simulink model "Likitha_Version_3_1"  (R2025b)
settings: Solver=VariableStepAuto  StartTime=0.0  StopTime=0.3  RelTol=1e-3
undefined symbols (not defined in the file): Ion, Lithium
libraries: spsBatteryLib x50, spsSeriesRLCBranchLib x15, spsCurrentMeasurementLib x10, spsVoltageMeasurementLib x10, spsIdealSwitchLib x9, spsMosfetLib x7, slpidlib x4, spsPWMGeneratorDCDCLib x2, spspowerguiLib x2, spsACVoltageSourceLib x1, eeHysteresisControl x1, spsDCMachineLib x1
(part 1 of 3)
settings Model: Creator=Jatay  LastModifiedBy=Jatay

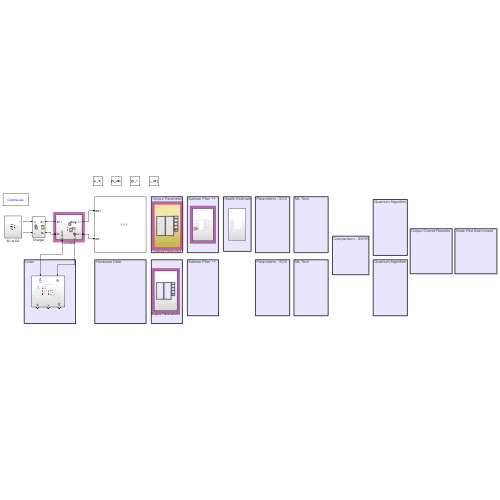
[thumbnail: Simulink's stored preview of the top-level diagram]
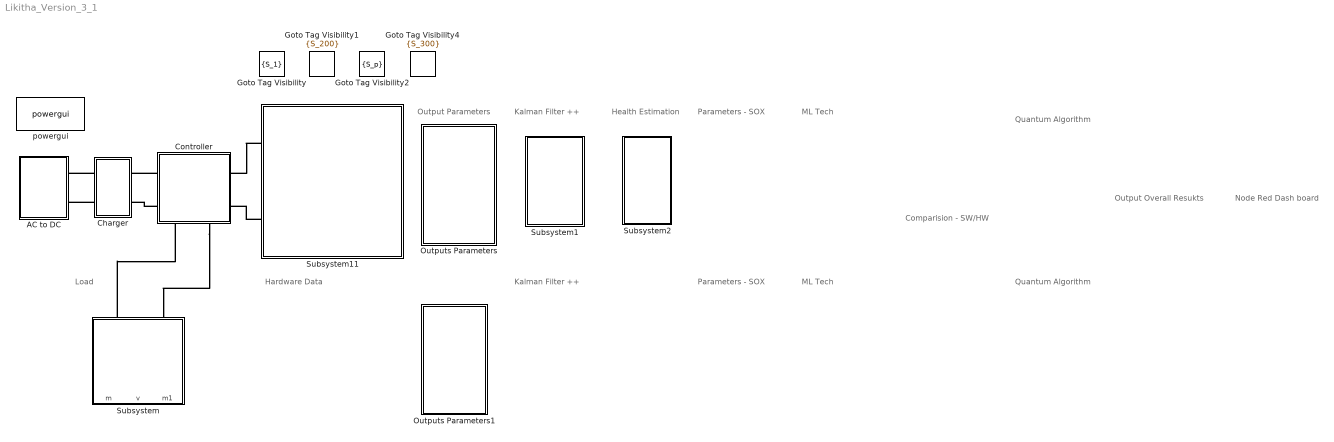
== system Likitha_Version_3_1 ==
  note: Health Estimation
  note: Output Parameters
  note: Hardware Data
  note: Kalman Filter ++
  note: Parameters - SOX
  note: ML Tech
  note: Kalman Filter ++
  note: Parameters - SOX
  note: ML Tech
  note: Comparision - SW/HW
  note: Quantum Algorithm
  note: Quantum Algorithm
  note: Output Overall Resukts
  note: Node Red Dash board
  note: Load
  AC to DC : Subsystem
  Charger : Subsystem
  Controller : Subsystem
      settings: PortSchema="{\"entries\":[{\"content\":{\"sides\":[{\"content\":{\"connectorIds\":[\"LConn1\",\"LConn2\"]},\"type\":\"ConnectorPlacement.EquallySpacedRectSide\",\"uuid\":\"ff826bc9-6c6d-4d1b-bda7-2b84bf27e69f\"},{\"content\":{\"connectorIds\":[\"RConn1\",\"RConn2\"],\"side\":\"RIGHT\"},\"type\":\"ConnectorPlacement.EquallySpacedRectSide\",\"uuid\":\"011d9e86-4a41-4c7c-aeec-abd747732ee3\"},{\"content\":{\"side\":\"TOP\"},\"type\":\"ConnectorPlacement.EquallySpacedRectSide\",\"uuid\":\"d78c1a77-7558-4fb8-9c60-436806204744\"},{\"content\":{\"connectorIds\":[\"RConn3\",\"RConn4\"],\"side\":\"BOTTOM\"},\"type\":\"ConnectorPlacement.EquallySpacedRectSide\",\"uuid\":\"cc43dd25-8365-4f89-92e1-f58595e4ba76\"}]},\"type\":\"ConnectorPlacement.EquallySpacedConnector\",\"uuid\":\"01dac08a-c3c2-418e-8901-b9ec60af109b\"}],\"packageUris\":[\"http://schema.mathworks.com/mf0/Connector/R2020b\"],\"version\":\"1.0\"}"
  Goto Tag Visibility : GotoTagVisibility  GotoTag=S_1
  Goto Tag Visibility1 : GotoTagVisibility  GotoTag=S_200
  Goto Tag Visibility2 : GotoTagVisibility  GotoTag=S_p
  Goto Tag Visibility4 : GotoTagVisibility  GotoTag=S_300
  Outputs Parameters : Subsystem
  Outputs Parameters1 : Subsystem
  Subsystem : Subsystem
  Subsystem1 : Subsystem
  Subsystem11 : Subsystem
      mask Display: image('swapping.webp');
  Subsystem2 : Subsystem
  powergui : spspowerguiLib/powergui  Priority=1  SimulationMode=Continuous  SampleTime=50e-6  frequency=60  Iterations=50  frequencyindice=0  Pbase=100e6  ErrMax=1e-4  UnitsV=kV  UnitsW=MW  buscounter=0  FunctionMessages=off  echomessages=off  EnableUseOfTLC=off  CurrentSourceSwitches=off  DisableSnubberDevices=off  DisableRonSwitches=off  DisableVfSwitches=off  DisplayEquations=off  AutomaticDiscreteSolvers=off  SolverType=Tustin/Backward Euler (TBE)  Interpol=off  ExternalGateDelay=off  methode=off  Ts=100  x0status=blocks  SPID=on  SwTol=0  HookPort=off  NonlinearTolerance=1e-4  nMaxIteration=100  ContinueOnMaxIteration=off  RestoreLinks=warning  ResistiveCurrentMeasurement=off  Frange=[0:2:500]  Ylog=off  Xlog=on  ShowGrid=off  save=off  variable=ZData  structure=0  ZoomFFT=off  StartTime=0.0  cycles=1  DisplayStyle=1  fundamental=60  FreqAxis=off  MaxFrequency=1000  frequencyindicesteady=1  RmsSteady=1  display=off
  connections:
  Charger/LConn1 -- AC to DC/RConn1
  Charger/LConn2 -- AC to DC/RConn2
  Controller/LConn1 -- Charger/RConn1
  Controller/LConn2 -- Charger/RConn2
  Subsystem11/LConn1 -- Controller/RConn1
  Subsystem11/LConn2 -- Controller/RConn2
  Subsystem/LConn1 -- Controller/RConn3
  Controller/RConn4 -- Subsystem/LConn2

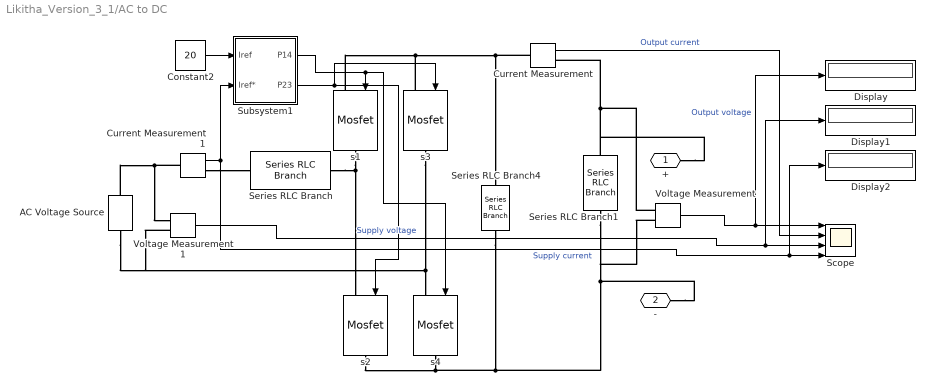
== system Likitha_Version_3_1/AC to DC ==
  AC Voltage Source : spsACVoltageSourceLib/AC Voltage Source  Amplitude=230*sqrt(2)  Phase=0  Frequency=50  SampleTime=0  Measurements=None  BusType=swing  Pref=10e3  Qref=0  Qmin=-inf  Qmax=+inf
  Constant2 : Constant  Value=20
  Current Measurement : spsCurrentMeasurementLib/Current Measurement  PhasorSimulation=off  OutputType=Complex  PSBequivalent=0
  Current Measurement1 : spsCurrentMeasurementLib/Current Measurement  PhasorSimulation=off  OutputType=Complex  PSBequivalent=0
  Display : Display
  Display1 : Display
      settings: Format=short_e
  Display2 : Display
  Scope : Scope  NumInputPorts=4
      settings: ActiveDisplayYMinimum=0  ActiveDisplayYMaximum=500
  Series RLC Branch : spsSeriesRLCBranchLib/Series RLC Branch  LConnTagsString=__new0  RConnTagsString=__new0  BranchType=L  Resistance=1  Inductance=10e-3  SetiL0=off  InitialCurrent=0  Capacitance=1e-6  Setx0=off  InitialVoltage=0  Measurements=None
  Series RLC Branch1 : spsSeriesRLCBranchLib/Series RLC Branch  LConnTagsString=__new0  RConnTagsString=__new0  BranchType=R  Resistance=1  Inductance=10e-3  SetiL0=off  InitialCurrent=0  Capacitance=1e-6  Setx0=off  InitialVoltage=0  Measurements=None
  Series RLC Branch4 : spsSeriesRLCBranchLib/Series RLC Branch  LConnTagsString=__new0  RConnTagsString=__new0  BranchType=C  Resistance=1  Inductance=1e-3  SetiL0=off  InitialCurrent=0  Capacitance=5000e-6  Setx0=off  InitialVoltage=0  Measurements=None
  Subsystem1 : Subsystem
  Voltage Measurement : spsVoltageMeasurementLib/Voltage Measurement  PhasorSimulation=off  OutputType=Complex  PSBequivalent=0
  Voltage Measurement1 : spsVoltageMeasurementLib/Voltage Measurement  PhasorSimulation=off  OutputType=Complex  PSBequivalent=0
  s{1..4} (4 alike) : spsMosfetLib/Mosfet  Ron=0.1  Lon=0  Rd=0.01  Vfd=0  IC=0  Rs=1e5  Cs=inf  Measurements=off
  + : PMIOPort  Side=Right
  - : PMIOPort  Port=2  Side=Right
  wires:
  Current Measurement1/1 -> Display2/1, Scope/4, Subsystem1/2(Iref*)  "Supply current"
  Voltage Measurement/1 -> Display/1, Scope/1  "Output voltage"
  Voltage Measurement1/1 -> Display1/1, Scope/3  "Supply voltage"
  Subsystem1/1("P14 ") -> s4/1, s1/1
  Current Measurement/1 -> Scope/2  "Output current"
  Subsystem1/2(P23) -> s3/1, s2/1
  Constant2/1 -> Subsystem1/1(Iref)
  connections:
  Current Measurement1/LConn1 -- Voltage Measurement1/LConn1 -- AC Voltage Source/RConn1
  Voltage Measurement/LConn1 -- Current Measurement/RConn1 -- Series RLC Branch1/LConn1 -- +/RConn1
  s3/RConn1 -- AC Voltage Source/LConn1 -- Voltage Measurement1/LConn2 -- s4/LConn1
  s2/RConn1 -- s4/RConn1 -- Series RLC Branch4/RConn1 -- Series RLC Branch1/RConn1 -- Voltage Measurement/LConn2 -- -/RConn1
  s1/RConn1 -- s2/LConn1 -- Series RLC Branch/RConn1
  s1/LConn1 -- Current Measurement/LConn1 -- Series RLC Branch4/LConn1 -- s3/LConn1
  Current Measurement1/RConn1 -- Series RLC Branch/LConn1

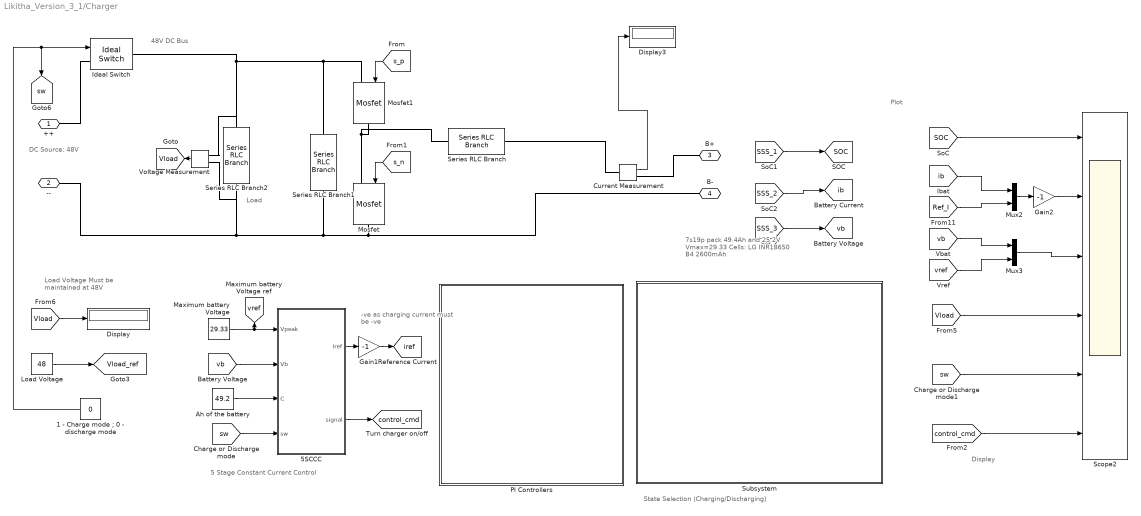
== system Likitha_Version_3_1/Charger ==
  note: Load Voltage
      | Must be
      | maintained at 48V
  note: 48V DC Bus
  note: DC Source:
      | 48V
  note: 7s19p pack
      | 49.4Ah and 25.2V
      | Vmax=29.33
      | Cells:
      | LG INR18650 B4 2600mAh
  note: Plot
  note: -ve as charging
      | current must be -ve
  note: 5 Stage Constant Current Control
  note: Display
  note: Load
  note: State Selection (Charging/Discharging)
  "1 - Charge mode ; 0 - discharge mode  " : Constant  Value=0
  5SCCC : Stateflow chart  TreatAsAtomicUnit=on
  Ah of the battery : Constant  Value=49.2
  Current Measurement : spsCurrentMeasurementLib/Current Measurement  PhasorSimulation=off  OutputType=Complex  PSBequivalent=0
  Display : Display
  Display3 : Display
  Gain1 : Gain  Gain=-1
  Gain2 : Gain  Gain=-1
  Ideal Switch : spsIdealSwitchLib/Ideal Switch  Ron=0.001  Lon=0  IC=0  Rs=1e5  Cs=inf  Measurements=off
  Load Voltage : Constant  Value=48
  Maximum battery Voltage : Constant  Value=29.33
  Mosfet : spsMosfetLib/Mosfet  Ron=0.1  Lon=0  Rd=0.01  Vfd=0  IC=0  Rs=1e5  Cs=inf  Measurements=off
  Mosfet1 : spsMosfetLib/Mosfet  Ron=0.1  Lon=0  Rd=0.01  Vfd=0  IC=0  Rs=1e5  Cs=inf  Measurements=off
  Mux2 : Mux  Inputs=2
  Mux3 : Mux  Inputs=2
  PI Controllers : Subsystem
  Scope2 : Scope  NumInputPorts=6
      settings: Title=SoC  ActiveDisplayYMinimum=96.96249  ActiveDisplayYMaximum=97.0551  DataLoggingVariableName=ScopeData2
  Series RLC Branch : spsSeriesRLCBranchLib/Series RLC Branch  LConnTagsString=__new0  RConnTagsString=__new0  BranchType=RL  Resistance=0.05  Inductance=5.76e-4  SetiL0=off  InitialCurrent=0  Capacitance=1e-6  Setx0=off  InitialVoltage=0  Measurements=None
  Series RLC Branch1 : spsSeriesRLCBranchLib/Series RLC Branch  LConnTagsString=__new0  RConnTagsString=__new0  BranchType=RC  Resistance=0.001  Inductance=5.76e-4  SetiL0=off  InitialCurrent=0  Capacitance=1000e-6  Setx0=off  InitialVoltage=0  Measurements=None
  Series RLC Branch2 : spsSeriesRLCBranchLib/Series RLC Branch  LConnTagsString=__new0  RConnTagsString=__new0  BranchType=R  Resistance=6  Inductance=5.76e-4  SetiL0=off  InitialCurrent=0  Capacitance=1000e-6  Setx0=off  InitialVoltage=0  Measurements=None
  Subsystem : Subsystem
  Voltage Measurement : spsVoltageMeasurementLib/Voltage Measurement  PhasorSimulation=off  OutputType=Complex  PSBequivalent=0
  ++ : PMIOPort  Side=Left
  -- : PMIOPort  Port=2  Side=Left
  B+ : PMIOPort  Port=3  Side=Right
  B- : PMIOPort  Port=4  Side=Right
  tag scope: SOC=global, Vload=global, Vload_ref=global, control_cmd=global, ib=global, iref=global, sw=global, vb=global, vref=global
  wires:
  Maximum battery Voltage/1 -> 5SCCC/1(Vpeak), [vref]
  [SSS_2] -> [ib]
  [s_n] -> Mosfet/1
  Mux3/1 -> Scope2/3
  [sw] -> Scope2/5
  Current Measurement/1 -> Display3/1
  Ah of the battery/1 -> 5SCCC/3(C)
  Mux2/1 -> Gain2/1
  Gain1/1 -> [iref]
  Gain2/1 -> Scope2/2
  [vb] -> 5SCCC/2(Vb)
  [SOC] -> Scope2/1
  Load Voltage/1 -> [Vload_ref]
  [SSS_3] -> [vb]
  [Ref_I] -> Mux2/2
  [control_cmd] -> Scope2/6
  [s_p] -> Mosfet1/1
  [Vload] -> Scope2/4
  [Vload] -> Display/1
  [vref] -> Mux3/2
  [vb] -> Mux3/1
  Voltage Measurement/1 -> [Vload]
  [sw] -> 5SCCC/4(sw)
  [ib] -> Mux2/1
  5SCCC/2(signal) -> [control_cmd]
  "1 - Charge mode ; 0 - discharge mode  "/1 -> Ideal Switch/1, [sw]
  [SSS_1] -> [SOC]
  5SCCC/1(Iref) -> Gain1/1
  connections:
  ++/RConn1 -- Ideal Switch/LConn1
  --/RConn1 -- Series RLC Branch2/RConn1 -- Voltage Measurement/LConn2 -- Series RLC Branch1/RConn1 -- B-/RConn1 -- Mosfet/RConn1
  Mosfet1/RConn1 -- Series RLC Branch/LConn1 -- Mosfet/LConn1
  Series RLC Branch1/LConn1 -- Voltage Measurement/LConn1 -- Series RLC Branch2/LConn1 -- Ideal Switch/RConn1 -- Mosfet1/LConn1
  B+/RConn1 -- Current Measurement/RConn1
  Series RLC Branch/RConn1 -- Current Measurement/LConn1

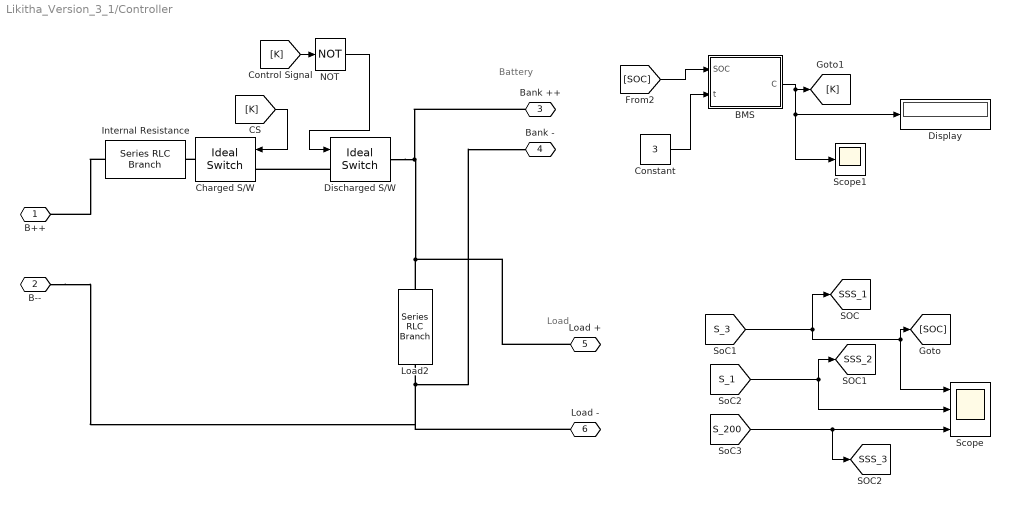
== system Likitha_Version_3_1/Controller ==
  note: Battery
  note: Load
  BMS : MATLAB Function  TreatAsAtomicUnit=on
  Charged S/W : spsIdealSwitchLib/Ideal Switch  Ron=0.001  Lon=0  IC=0  Rs=1e5  Cs=inf  Measurements=off
  Constant : Constant  Value=3
  Discharged S/W : spsIdealSwitchLib/Ideal Switch  Ron=0.001  Lon=0  IC=0  Rs=1e5  Cs=inf  Measurements=off
  Display : Display
  Internal Resistance : spsSeriesRLCBranchLib/Series RLC Branch  LConnTagsString=__new0  RConnTagsString=__new0  BranchType=R  Resistance=0.01  Inductance=1e-3  SetiL0=off  InitialCurrent=0  Capacitance=1e-6  Setx0=off  InitialVoltage=0  Measurements=None
  Load2 : spsSeriesRLCBranchLib/Series RLC Branch  LConnTagsString=__new0  RConnTagsString=__new0  BranchType=R  Resistance=1  Inductance=1e-3  SetiL0=off  InitialCurrent=0  Capacitance=1e-6  Setx0=off  InitialVoltage=0  Measurements=None
  NOT : Logic  Operator=NOT  IconShape=distinctive  AllPortsSameDT=off  OutDataTypeStr=boolean
  Scope : Scope  NumInputPorts=3
      settings: ActiveDisplayYMinimum=3910.04343  ActiveDisplayYMaximum=3910.05965
  Scope1 : Scope
      settings: ActiveDisplayYMinimum=0.9  ActiveDisplayYMaximum=1.1
  B++ : PMIOPort  Side=Left
  B-- : PMIOPort  Port=2  Side=Left
  Bank ++ : PMIOPort  Port=3  Side=Right
  Bank - : PMIOPort  Port=4  Side=Right
  Load + : PMIOPort  Port=5  Side=Right
  Load - : PMIOPort  Port=6  Side=Right
  tag scope: SSS_1=global, SSS_2=global, SSS_3=global
  wires:
  [K] -> NOT/1
  NOT/1 -> Discharged S/W/1
  [S_3] -> Scope/1, [SOC], [SSS_1]
  [K] -> Charged S/W/1
  [S_1] -> Scope/2, [SSS_2]
  [SOC] -> BMS/1(SOC)
  BMS/1(C) -> Scope1/1, Display/1, [K]
  [S_200] -> [SSS_3], Scope/3
  Constant/1 -> BMS/2(t)
  connections:
  Charged S/W/RConn1 -- Internal Resistance/LConn1
  Internal Resistance/RConn1 -- B++/RConn1
  Discharged S/W/RConn1 -- Bank ++/RConn1 -- Load2/LConn1 -- Load +/RConn1
  Load -/RConn1 -- B--/RConn1 -- Load2/RConn1 -- Bank -/RConn1
  Discharged S/W/LConn1 -- Charged S/W/LConn1

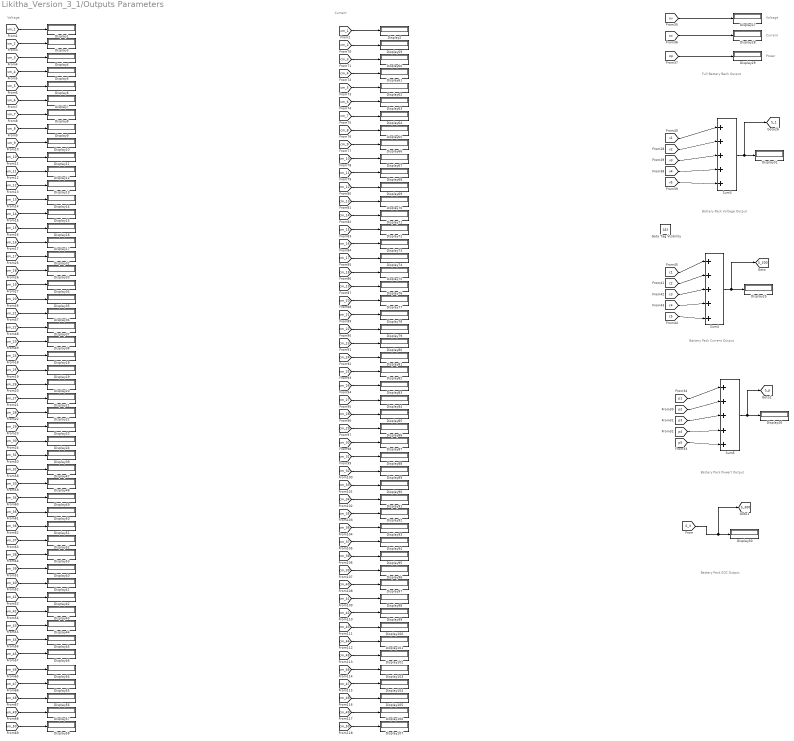
== system Likitha_Version_3_1/Outputs Parameters ==
  note: Voltage
  note: Full Battery Bank Output
  note: Voltage
  note: Current
  note: Power
  note: Battery Pack Voltage Output
  note: Battery Pack Current Output
  note: Battery Pack Powert Output
  note: Battery Pack SOC Output
  note: Current
  Display{1..107} (107 alike) : Display
  Goto Tag Visibility : GotoTagVisibility
  Sum3 : Sum  Inputs=|+++++
  Sum4 : Sum  Inputs=|+++++
  Sum5 : Sum  Inputs=|+++++
  tag scope: S_1=global, S_200=global, S_300=global, S_p=global
  wires:
  [ov] -> Display27/1
  [op] -> Display29/1
  Sum4/1 -> [S_200], Display25/1
  [v3] -> Sum3/3
  [p2] -> Sum5/2
  [v2] -> Sum3/2
  [c4] -> Sum4/4
  [v1] -> Sum3/1
  [c2] -> Sum4/2
  [v4] -> Sum3/4
  [p5] -> Sum5/5
  [c3] -> Sum4/3
  [p3] -> Sum5/3
  Sum3/1 -> [S_1], Display31/1
  [p1] -> Sum5/1
  [oc] -> Display28/1
  [v5] -> Sum3/5
  [c5] -> Sum4/5
  [p4] -> Sum5/4
  [c1] -> Sum4/1
  Sum5/1 -> [S_p], Display26/1
  [vm_1] -> Display1/1
  [cm_1] -> Display2/1
  [vm_2] -> Display3/1
  [vm_3] -> Display4/1
  [vm_4] -> Display5/1
  [vm_5] -> Display6/1
  [vm_8] -> Display9/1
  [vm_9] -> Display10/1
  [vm_10] -> Display11/1
  [vm_7] -> Display8/1
  [vm_6] -> Display7/1
  [vm_13] -> Display14/1
  [vm_14] -> Display15/1
  [vm_15] -> Display16/1
  [vm_12] -> Display13/1
  [vm_11] -> Display12/1
  [vm_18] -> Display33/1
  [vm_24] -> Display18/1
  [vm_21] -> Display36/1
  [vm_22] -> Display37/1
  [vm_25] -> Display19/1
  [vm_23] -> Display38/1
  [vm_19] -> Display34/1
  [vm_20] -> Display35/1
  [vm_30] -> Display24/1
  [vm_26] -> Display20/1
  [vm_27] -> Display21/1
  [vm_17] -> Display32/1
  [vm_29] -> Display23/1
  [vm_16] -> Display17/1
  [vm_28] -> Display22/1
  [vm_33] -> Display48/1
  [vm_39] -> Display40/1
  [vm_36] -> Display51/1
  [vm_37] -> Display52/1
  [vm_40] -> Display41/1
  [vm_38] -> Display53/1
  [vm_34] -> Display49/1
  [vm_35] -> Display50/1
  [vm_45] -> Display46/1
  [vm_41] -> Display42/1
  [vm_42] -> Display43/1
  [vm_32] -> Display47/1
  [vm_44] -> Display45/1
  [vm_31] -> Display39/1
  [vm_43] -> Display44/1
  [vm_47] -> Display55/1
  [vm_46] -> Display54/1
  [vm_50] -> Display58/1
  [vm_48] -> Display56/1
  [vm_49] -> Display57/1
  [cm_2] -> Display59/1
  [cm_3] -> Display60/1
  [cm_4] -> Display61/1
  [cm_5] -> Display62/1
  [cm_9] -> Display66/1
  [cm_6] -> Display63/1
  [cm_10] -> Display67/1
  [cm_8] -> Display65/1
  [cm_7] -> Display64/1
  [cm_19] -> Display76/1
  [cm_18] -> Display75/1
  [cm_20] -> Display77/1
  [cm_17] -> Display74/1
  [cm_14] -> Display71/1
  [cm_11] -> Display68/1
  [cm_15] -> Display72/1
  [cm_13] -> Display70/1
  [cm_12] -> Display69/1
  [cm_16] -> Display73/1
  [cm_29] -> Display86/1
  [cm_28] -> Display85/1
  [cm_30] -> Display87/1
  [cm_27] -> Display84/1
  [cm_24] -> Display81/1
  [cm_21] -> Display78/1
  [cm_25] -> Display82/1
  [cm_23] -> Display80/1
  [cm_22] -> Display79/1
  [cm_26] -> Display83/1
  [cm_39] -> Display96/1
  [cm_38] -> Display95/1
  [cm_40] -> Display97/1
  [cm_37] -> Display94/1
  [cm_34] -> Display91/1
  [cm_31] -> Display88/1
  [cm_35] -> Display92/1
  [cm_33] -> Display90/1
  [cm_32] -> Display89/1
  [cm_36] -> Display93/1
  [cm_49] -> Display106/1
  [cm_48] -> Display105/1
  [cm_50] -> Display107/1
  [cm_47] -> Display104/1
  [cm_44] -> Display101/1
  [cm_41] -> Display98/1
  [cm_45] -> Display102/1
  [cm_43] -> Display100/1
  [cm_42] -> Display99/1
  [cm_46] -> Display103/1
  [S_3] -> [S_300], Display30/1

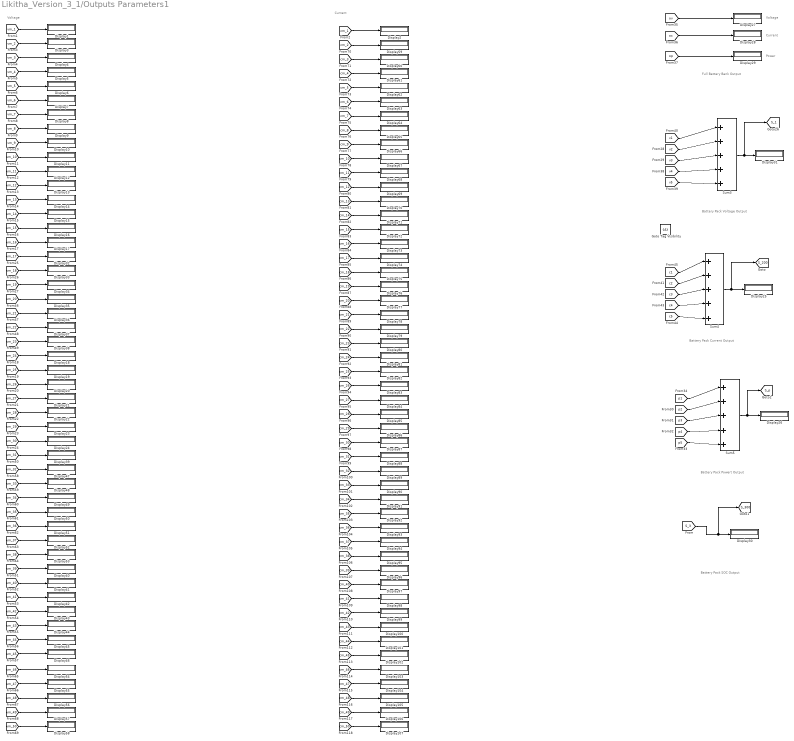
== system Likitha_Version_3_1/Outputs Parameters1 ==
  note: Voltage
  note: Full Battery Bank Output
  note: Voltage
  note: Current
  note: Power
  note: Battery Pack Voltage Output
  note: Battery Pack Current Output
  note: Battery Pack Powert Output
  note: Battery Pack SOC Output
  note: Current
  Display{1..107} (107 alike) : Display
  Goto Tag Visibility : GotoTagVisibility
  Sum3 : Sum  Inputs=|+++++
  Sum4 : Sum  Inputs=|+++++
  Sum5 : Sum  Inputs=|+++++
  tag scope: S_1=global, S_200=global, S_300=global, S_p=global
  wires:
  [ov] -> Display27/1
  [op] -> Display29/1
  Sum4/1 -> [S_200], Display25/1
  [v3] -> Sum3/3
  [p2] -> Sum5/2
  [v2] -> Sum3/2
  [c4] -> Sum4/4
  [v1] -> Sum3/1
  [c2] -> Sum4/2
  [v4] -> Sum3/4
  [p5] -> Sum5/5
  [c3] -> Sum4/3
  [p3] -> Sum5/3
  Sum3/1 -> [S_1], Display31/1
  [p1] -> Sum5/1
  [oc] -> Display28/1
  [v5] -> Sum3/5
  [c5] -> Sum4/5
  [p4] -> Sum5/4
  [c1] -> Sum4/1
  Sum5/1 -> [S_p], Display26/1
  [vm_1] -> Display1/1
  [cm_1] -> Display2/1
  [vm_2] -> Display3/1
  [vm_3] -> Display4/1
  [vm_4] -> Display5/1
  [vm_5] -> Display6/1
  [vm_8] -> Display9/1
  [vm_9] -> Display10/1
  [vm_10] -> Display11/1
  [vm_7] -> Display8/1
  [vm_6] -> Display7/1
  [vm_13] -> Display14/1
  [vm_14] -> Display15/1
  [vm_15] -> Display16/1
  [vm_12] -> Display13/1
  [vm_11] -> Display12/1
  [vm_18] -> Display33/1
  [vm_24] -> Display18/1
  [vm_21] -> Display36/1
  [vm_22] -> Display37/1
  [vm_25] -> Display19/1
  [vm_23] -> Display38/1
  [vm_19] -> Display34/1
  [vm_20] -> Display35/1
  [vm_30] -> Display24/1
  [vm_26] -> Display20/1
  [vm_27] -> Display21/1
  [vm_17] -> Display32/1
  [vm_29] -> Display23/1
  [vm_16] -> Display17/1
  [vm_28] -> Display22/1
  [vm_33] -> Display48/1
  [vm_39] -> Display40/1
  [vm_36] -> Display51/1
  [vm_37] -> Display52/1
  [vm_40] -> Display41/1
  [vm_38] -> Display53/1
  [vm_34] -> Display49/1
  [vm_35] -> Display50/1
  [vm_45] -> Display46/1
  [vm_41] -> Display42/1
  [vm_42] -> Display43/1
  [vm_32] -> Display47/1
  [vm_44] -> Display45/1
  [vm_31] -> Display39/1
  [vm_43] -> Display44/1
  [vm_47] -> Display55/1
  [vm_46] -> Display54/1
  [vm_50] -> Display58/1
  [vm_48] -> Display56/1
  [vm_49] -> Display57/1
  [cm_2] -> Display59/1
  [cm_3] -> Display60/1
  [cm_4] -> Display61/1
  [cm_5] -> Display62/1
  [cm_9] -> Display66/1
  [cm_6] -> Display63/1
  [cm_10] -> Display67/1
  [cm_8] -> Display65/1
  [cm_7] -> Display64/1
  [cm_19] -> Display76/1
  [cm_18] -> Display75/1
  [cm_20] -> Display77/1
  [cm_17] -> Display74/1
  [cm_14] -> Display71/1
  [cm_11] -> Display68/1
  [cm_15] -> Display72/1
  [cm_13] -> Display70/1
  [cm_12] -> Display69/1
  [cm_16] -> Display73/1
  [cm_29] -> Display86/1
  [cm_28] -> Display85/1
  [cm_30] -> Display87/1
  [cm_27] -> Display84/1
  [cm_24] -> Display81/1
  [cm_21] -> Display78/1
  [cm_25] -> Display82/1
  [cm_23] -> Display80/1
  [cm_22] -> Display79/1
  [cm_26] -> Display83/1
  [cm_39] -> Display96/1
  [cm_38] -> Display95/1
  [cm_40] -> Display97/1
  [cm_37] -> Display94/1
  [cm_34] -> Display91/1
  [cm_31] -> Display88/1
  [cm_35] -> Display92/1
  [cm_33] -> Display90/1
  [cm_32] -> Display89/1
  [cm_36] -> Display93/1
  [cm_49] -> Display106/1
  [cm_48] -> Display105/1
  [cm_50] -> Display107/1
  [cm_47] -> Display104/1
  [cm_44] -> Display101/1
  [cm_41] -> Display98/1
  [cm_45] -> Display102/1
  [cm_43] -> Display100/1
  [cm_42] -> Display99/1
  [cm_46] -> Display103/1
  [S_3] -> [S_300], Display30/1

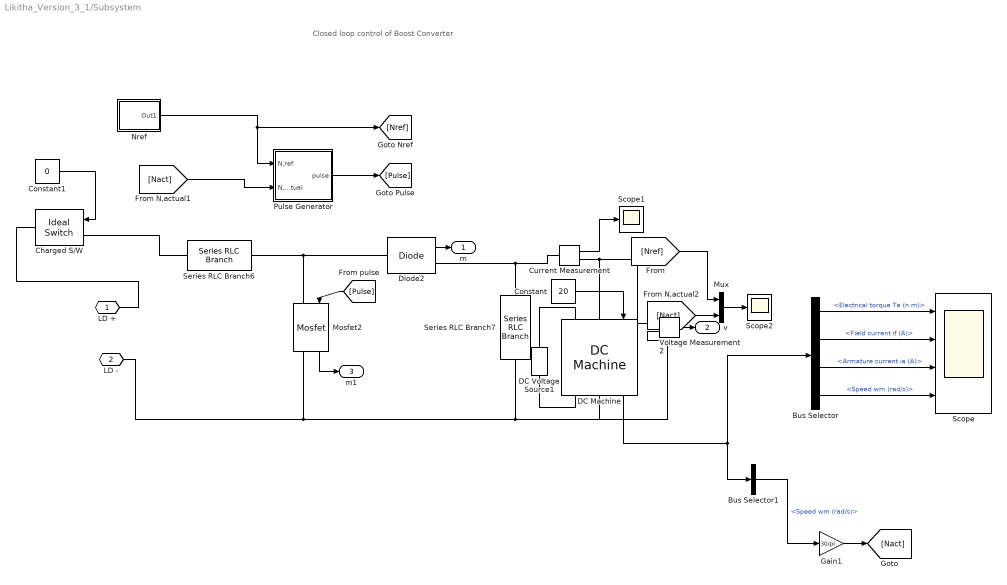
== system Likitha_Version_3_1/Subsystem ==
  note: Closed loop control of Boost Converter
  Bus Selector : BusSelector  OutputSignals=Electrical torque Te (n m),Field current if (A),Armature current ia (A),Speed wm (rad/s)
  Bus Selector1 : BusSelector  OutputSignals=Speed wm (rad/s)
  Charged S/W : spsIdealSwitchLib/Ideal Switch  Ron=0.001  Lon=0  IC=0  Rs=1e5  Cs=inf  Measurements=off
  Constant : Constant  Value=20
  Constant1 : Constant  Value=0
  Current Measurement : spsCurrentMeasurementLib/Current Measurement  PhasorSimulation=off  OutputType=Complex  PSBequivalent=0
  DC Machine : spsDCMachineLib/DC Machine  PresetModel=No  MechanicalLoad=Torque TL  FieldType=Wound  ShowDetailedParameters=on  MeasurementBus=off  RLa=[2.581 0.0058]  RLf=[281.3 156]  Laf=0.9483  MachineConstant=Torque constant (N.m/A)  Ke=1.8  Kt=1.8  J=0.02215  Bm=0.002953  Tf=0.5161  w0=0  Ifinit=0.853181656594383  TsPowergui=0  TsBlock=-1
  DC Voltage Source1 : spsDCVoltageSourceLib/DC Voltage Source  Amplitude=240  Measurements=None
  Diode2 : spsDiodeLib/Diode  Ron=0.001  Lon=0  Vf=0.8  IC=0  UseSnubber=off  Rs=500  Cs=250e-9  Measurements=on
  Gain1 : Gain  Gain=30/pi
  Mosfet2 : spsMosfetLib/Mosfet  Ron=0.1  Lon=0  Rd=0.01  Vfd=0  IC=0  Rs=1e5  Cs=inf  Measurements=on
  Mux : Mux  Inputs=2
  Nref : Subsystem
  Pulse Generator : Subsystem
  Scope : Scope  NumInputPorts=4
      settings: ActiveDisplayYMinimum=-2.2358069715761362  ActiveDisplayYMaximum=20.122262744185228  DataLoggingVariableName=ScopeData3
  Scope1 : Scope
      settings: ActiveDisplayYMinimum=-62.50723  ActiveDisplayYMaximum=562.55999
  Scope2 : Scope
      settings: ActiveDisplayYMinimum=-156.12988  ActiveDisplayYMaximum=1251.48302
  Series RLC Branch6 : spsSeriesRLCBranchLib/Series RLC Branch  LConnTagsString=__new0  RConnTagsString=__new0  BranchType=L  Resistance=1  Inductance=1e-4  SetiL0=off  InitialCurrent=0  Capacitance=1e-6  Setx0=off  InitialVoltage=0  Measurements=None
  Series RLC Branch7 : spsSeriesRLCBranchLib/Series RLC Branch  LConnTagsString=__new0  RConnTagsString=__new0  BranchType=C  Resistance=1  Inductance=5e-4  SetiL0=off  InitialCurrent=0  Capacitance=30e-4  Setx0=off  InitialVoltage=0  Measurements=None
  Voltage Measurement2 : spsVoltageMeasurementLib/Voltage Measurement  PhasorSimulation=off  OutputType=Complex  PSBequivalent=0
  LD + : PMIOPort  Side=Left
  LD - : PMIOPort  Port=2  Side=Left
  m : Outport
  v : Outport  Port=2
  m1 : Outport  Port=3
  wires:
  Nref/1(Out1) -> [Nref], Pulse Generator/1(N,ref)
  DC Machine/1 -> Bus Selector1/1, Bus Selector/1
  [Nref] -> Mux/1
  Voltage Measurement2/1 -> v/1
  [Nact] -> Mux/2
  Bus Selector1/1 -> Gain1/1  "<Speed wm (rad/s)>"
  Diode2/1 -> m/1
  [Pulse] -> Mosfet2/1
  Gain1/1 -> [Nact]
  [Nact] -> Pulse Generator/2(N,actual)
  Mosfet2/1 -> m1/1
  Pulse Generator/1(pulse) -> [Pulse]
  Current Measurement/1 -> Scope1/1
  Constant/1 -> DC Machine/1
  Mux/1 -> Scope2/1
  Bus Selector/1 -> Scope/1  "<Electrical torque Te (n m)>"
  Bus Selector/2 -> Scope/2  "<Field current if (A)>"
  Bus Selector/3 -> Scope/3  "<Armature current ia (A)>"
  Bus Selector/4 -> Scope/4  "<Speed wm (rad/s)>"
  Constant1/1 -> Charged S/W/1
  connections:
  DC Voltage Source1/LConn1 -- DC Machine/RConn2
  Series RLC Branch7/LConn1 -- Current Measurement/LConn1 -- Diode2/RConn1
  Current Measurement/RConn1 -- DC Machine/LConn1 -- Voltage Measurement2/LConn1
  Series RLC Branch7/RConn1 -- DC Machine/RConn1 -- Voltage Measurement2/LConn2 -- Mosfet2/RConn1 -- LD -/RConn1
  Diode2/LConn1 -- Mosfet2/LConn1 -- Series RLC Branch6/RConn1
  DC Voltage Source1/RConn1 -- DC Machine/LConn2
  Charged S/W/RConn1 -- LD +/RConn1
  Charged S/W/LConn1 -- Series RLC Branch6/LConn1

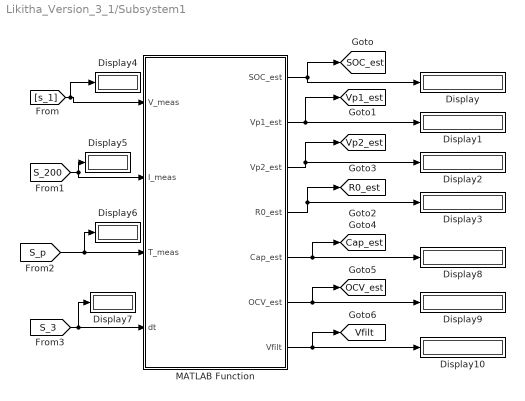
== system Likitha_Version_3_1/Subsystem1 ==
  Display{,1..10} (11 alike) : Display
  MATLAB Function : MATLAB Function  TreatAsAtomicUnit=on
  tag scope: Cap_est=global, OCV_est=global, R0_est=global, SOC_est=global, Vfilt=global, Vp1_est=global, Vp2_est=global
  wires:
  [S_p] -> Display6/1, MATLAB Function/3(T_meas)
  [S_3] -> Display7/1, MATLAB Function/4(dt)
  [s_1] -> MATLAB Function/1(V_meas), Display4/1
  [S_200] -> Display5/1, MATLAB Function/2(I_meas)
  MATLAB Function/1(SOC_est) -> [SOC_est], Display/1
  MATLAB Function/2(Vp1_est) -> [Vp1_est], Display1/1
  MATLAB Function/3(Vp2_est) -> Display2/1, [Vp2_est]
  MATLAB Function/4(R0_est) -> [R0_est], Display3/1
  MATLAB Function/5(Cap_est) -> [Cap_est], Display8/1
  MATLAB Function/6(OCV_est) -> [OCV_est], Display9/1
  MATLAB Function/7(Vfilt) -> [Vfilt], Display10/1

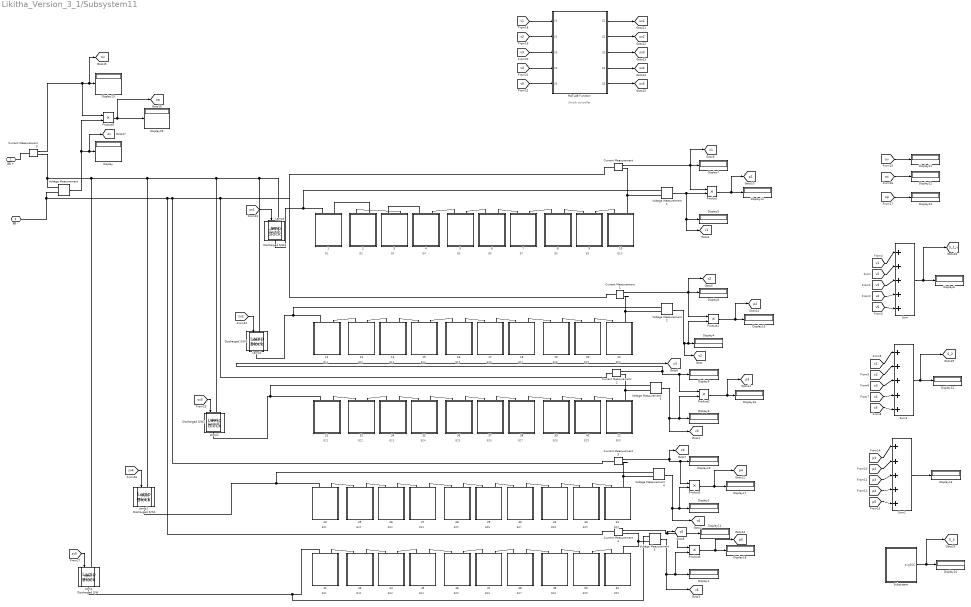
== system Likitha_Version_3_1/Subsystem11 ==
  note: Switch controller
  note: B1
  note: B2
  note: B3
  note: B4
  note: B6
  note: B5
  note: B7
  note: B9
  note: B8
  note: B11
  note: B18
  note: B17
  note: B13
  note: B15
  note: B19
  note: B16
  note: B12
  note: B14
  note: B10
  note: B20
  note: B21
  note: B28
  note: B29
  note: B27
  note: B25
  note: B26
  note: B30
  note: B40
  note: B23
  note: B35
  note: B37
  note: B33
  note: B36
  note: B39
  note: B32
  note: B24
  note: B34
  note: B38
  note: B31
  note: B22
  note: B47
  note: B42
  note: B49
  note: B46
  note: B43
  note: B44
  note: B41
  note: B45
  note: B48
  note: B50
  1 : Subsystem
      mask Display: image('sibgle battery.jpg');
  10 : Subsystem
      mask Display: image('sibgle battery.jpg');
  11 : Subsystem
      mask Display: image('sibgle battery.jpg');
  12 : Subsystem
      mask Display: image('sibgle battery.jpg');
  13 : Subsystem
      mask Display: image('sibgle battery.jpg');
  14 : Subsystem
      mask Display: image('sibgle battery.jpg');
  15 : Subsystem
      mask Display: image('sibgle battery.jpg');
  16 : Subsystem
      mask Display: image('sibgle battery.jpg');
  17 : Subsystem
      mask Display: image('sibgle battery.jpg');
  18 : Subsystem
      mask Display: image('sibgle battery.jpg');
  19 : Subsystem
      mask Display: image('sibgle battery.jpg');
  2 : Subsystem
      mask Display: image('sibgle battery.jpg');
  20 : Subsystem
      mask Display: image('sibgle battery.jpg');
  21 : Subsystem
      mask Display: image('sibgle battery.jpg');
  22 : Subsystem
      mask Display: image('sibgle battery.jpg');
  23 : Subsystem
      mask Display: image('sibgle battery.jpg');
  24 : Subsystem
      mask Display: image('sibgle battery.jpg');
  25 : Subsystem
      mask Display: image('sibgle battery.jpg');
  26 : Subsystem
      mask Display: image('sibgle battery.jpg');
  27 : Subsystem
      mask Display: image('sibgle battery.jpg');
  28 : Subsystem
      mask Display: image('sibgle battery.jpg');
  29 : Subsystem
      mask Display: image('sibgle battery.jpg');
  3 : Subsystem
      mask Display: image('sibgle battery.jpg');
  30 : Subsystem
      mask Display: image('sibgle battery.jpg');
  31 : Subsystem
      mask Display: image('sibgle battery.jpg');
  32 : Subsystem
      mask Display: image('sibgle battery.jpg');
  33 : Subsystem
      mask Display: image('sibgle battery.jpg');
  34 : Subsystem
      mask Display: image('sibgle battery.jpg');
  35 : Subsystem
      mask Display: image('sibgle battery.jpg');
  36 : Subsystem
      mask Display: image('sibgle battery.jpg');
  37 : Subsystem
      mask Display: image('sibgle battery.jpg');
  38 : Subsystem
      mask Display: image('sibgle battery.jpg');
  39 : Subsystem
      mask Display: image('sibgle battery.jpg');
  4 : Subsystem
      mask Display: image('sibgle battery.jpg');
  40 : Subsystem
      mask Display: image('sibgle battery.jpg');
  41 : Subsystem
      mask Display: image('sibgle battery.jpg');
  42 : Subsystem
      mask Display: image('sibgle battery.jpg');
  43 : Subsystem
      mask Display: image('sibgle battery.jpg');
  44 : Subsystem
      mask Display: image('sibgle battery.jpg');
  45 : Subsystem
      mask Display: image('sibgle battery.jpg');
  46 : Subsystem
      mask Display: image('sibgle battery.jpg');
  47 : Subsystem
      mask Display: image('sibgle battery.jpg');
  48 : Subsystem
      mask Display: image('sibgle battery.jpg');
  49 : Subsystem
      mask Display: image('sibgle battery.jpg');
  5 : Subsystem
      mask Display: image('sibgle battery.jpg');
  50 : Subsystem
      mask Display: image('sibgle battery.jpg');
  6 : Subsystem
      mask Display: image('sibgle battery.jpg');
  7 : Subsystem
      mask Display: image('sibgle battery.jpg');
  8 : Subsystem
      mask Display: image('sibgle battery.jpg');
  9 : Subsystem
      mask Display: image('sibgle battery.jpg');
  Current Measurement{,1..5} (6 alike) : spsCurrentMeasurementLib/Current Measurement  PhasorSimulation=off  OutputType=Complex  PSBequivalent=0
  Discharged S/W{,1..4} (5 alike) : spsIdealSwitchLib/Ideal Switch  Ron=0.001  Lon=0  IC=0  Rs=1e5  Cs=inf  Measurements=off
  Display{,1..24} (25 alike) : Display
      Display settings: Decimation=2
      Display11 settings: Decimation=3
      Display19 settings: Decimation=2
      Display20 settings: Decimation=2
  Lamp{,1..4} (5 alike) : LampBlock  LabelPosition=Hide  DefaultColor=[192.0, 192.0, 192.0]
  MATLAB Function : MATLAB Function  TreatAsAtomicUnit=on
  Product{,1..5} (6 alike) : Product
  Subsystem : Subsystem
  Sum : Sum  Inputs=|+++++
  Sum1 : Sum  Inputs=|+++++
  Sum2 : Sum  Inputs=|+++++
  Voltage Measurement{,1..5} (6 alike) : spsVoltageMeasurementLib/Voltage Measurement  PhasorSimulation=off  OutputType=Complex  PSBequivalent=0
  BB + : PMIOPort  Side=Left
  BB - : PMIOPort  Port=2  Side=Left
  tag scope: S_1_v=global, S_2=global, S_3=global, c1=global, c2=global, c3=global, c4=global, c5=global, oc=global, op=global, ov=global, p1=global, p2=global, p3=global, p4=global, p5=global, sv1=global, sv2=global, sv3=global, sv4=global, sv5=global, v1=global, v2=global, v3=global, v4=global, v5=global
  wires:
  Voltage Measurement/1 -> Product5/2, [oc], Display/1
  Voltage Measurement5/1 -> [v5], Product4/2, Display1/1
  Voltage Measurement4/1 -> [v4], Product3/2, Display2/1
  Voltage Measurement3/1 -> [v3], Product2/2, Display3/1
  Voltage Measurement2/1 -> [v2], Product1/2, Display4/1
  Voltage Measurement1/1 -> Display5/1, [v1], Product/2
  Sum/1 -> [S_1_v], Display6/1
  Current Measurement/1 -> Product/1, [c1], Display7/1
  Current Measurement1/1 -> Product1/1, [c2], Display8/1
  Current Measurement2/1 -> Product2/1, Display9/1, [c3]
  Current Measurement3/1 -> Product3/1, Display10/1, [c4]
  Current Measurement4/1 -> Product4/1, Display11/1, [c5]
  [v1] -> Sum/1
  [v2] -> Sum/2
  [v3] -> Sum/3
  [v4] -> Sum/4
  [v5] -> Sum/5
  Sum1/1 -> [S_2], Display12/1
  [c1] -> Sum1/1
  [c5] -> Sum1/5
  [c3] -> Sum1/3
  [c2] -> Sum1/2
  [c4] -> Sum1/4
  Product/1 -> [p1], Display14/1
  Product1/1 -> [p2], Display15/1
  Product2/1 -> [p3], Display16/1
  Product3/1 -> [p4], Display17/1
  Product4/1 -> [p5], Display18/1
  [p3] -> Sum2/3
  [p4] -> Sum2/4
  [p5] -> Sum2/5
  [p1] -> Sum2/1
  [p2] -> Sum2/2
  Sum2/1 -> Display13/1
  Current Measurement5/1 -> Product5/1, [ov], Display19/1
  Product5/1 -> [op], Display20/1
  [op] -> Display23/1
  [oc] -> Display22/1
  [ov] -> Display21/1
  Subsystem/1(avgSOC) -> [S_3], Display24/1
  [v1] -> MATLAB Function/1(V1)
  [v2] -> MATLAB Function/2(V2)
  [v3] -> MATLAB Function/3(V3)
  [v4] -> MATLAB Function/4(V4)
  [v5] -> MATLAB Function/5(V5)
  MATLAB Function/1(S1) -> [sv1]
  MATLAB Function/2(S2) -> [sv2]
  MATLAB Function/3(S3) -> [sv3]
  MATLAB Function/4(S4) -> [sv4]
  MATLAB Function/5(S5) -> [sv5]
  [sv1] -> Discharged S/W4/1
  [sv2] -> Discharged S/W3/1
  [sv3] -> Discharged S/W2/1
  [sv4] -> Discharged S/W1/1
  [sv5] -> Discharged S/W/1
  connections:
  Voltage Measurement/LConn1 -- Current Measurement5/RConn1 -- Discharged S/W/LConn1 -- Discharged S/W1/LConn1 -- Discharged S/W2/LConn1 -- Discharged S/W3/LConn1 -- Discharged S/W4/LConn1
  Voltage Measurement/LConn2 -- Current Measurement4/LConn1 -- Current Measurement3/LConn1 -- Current Measurement2/LConn1 -- Current Measurement/LConn1 -- Current Measurement1/LConn1 -- BB -/RConn1
  1/RConn2 -- 2/RConn2
  2/RConn1 -- 3/RConn2
  4/RConn1 -- 3/RConn1
  5/RConn1 -- 4/RConn2
  6/RConn1 -- 5/RConn2
  6/RConn2 -- 7/RConn1
  8/RConn1 -- 7/RConn2
  8/RConn2 -- 9/RConn1
  10/RConn1 -- 9/RConn2
  13/RConn1 -- 11/RConn2
  14/RConn1 -- 13/RConn2
  14/RConn2 -- 15/RConn1
  16/RConn1 -- 15/RConn2
  16/RConn2 -- 17/RConn1
  17/RConn2 -- 18/RConn1
  18/RConn2 -- 19/RConn1
  19/RConn2 -- 20/RConn1
  20/RConn2 -- 12/RConn1
  21/RConn2 -- 32/RConn1
  34/RConn1 -- 32/RConn2
  34/RConn2 -- 35/RConn1
  35/RConn2 -- 36/RConn1
  36/RConn2 -- 37/RConn1
  37/RConn2 -- 38/RConn1
  38/RConn2 -- 39/RConn1
  39/RConn2 -- 40/RConn1
  40/RConn2 -- 22/RConn1
  23/RConn2 -- 25/RConn1
  25/RConn2 -- 26/RConn1
  26/RConn2 -- 27/RConn1
  27/RConn2 -- 28/RConn1
  28/RConn2 -- 29/RConn1
  29/RConn2 -- 30/RConn1
  30/RConn2 -- 31/RConn1
  31/RConn2 -- 33/RConn1
  33/RConn2 -- 24/RConn1
  41/RConn2 -- 43/RConn1
  43/RConn2 -- 44/RConn1
  45/RConn1 -- 44/RConn2
  45/RConn2 -- 46/RConn1
  47/RConn1 -- 46/RConn2
  48/RConn1 -- 47/RConn2
  48/RConn2 -- 49/RConn1
  49/RConn2 -- 50/RConn1
  42/RConn1 -- 50/RConn2
  Current Measurement/RConn1 -- 10/RConn2 -- Voltage Measurement1/LConn2
  Current Measurement1/RConn1 -- 12/RConn2 -- Voltage Measurement2/LConn2
  Current Measurement2/RConn1 -- Voltage Measurement3/LConn2 -- 22/RConn2
  Current Measurement3/RConn1 -- 24/RConn2 -- Voltage Measurement4/LConn2
  Current Measurement4/RConn1 -- Voltage Measurement5/LConn2 -- 42/RConn2
  Current Measurement5/LConn1 -- BB +/RConn1
  41/RConn1 -- Voltage Measurement5/LConn1 -- Discharged S/W/RConn1
  23/RConn1 -- Voltage Measurement4/LConn1 -- Discharged S/W1/RConn1
  21/RConn1 -- Voltage Measurement3/LConn1 -- Discharged S/W2/RConn1
  11/RConn1 -- Voltage Measurement2/LConn1 -- Discharged S/W3/RConn1
  Discharged S/W4/RConn1 -- Voltage Measurement1/LConn1 -- 1/RConn1

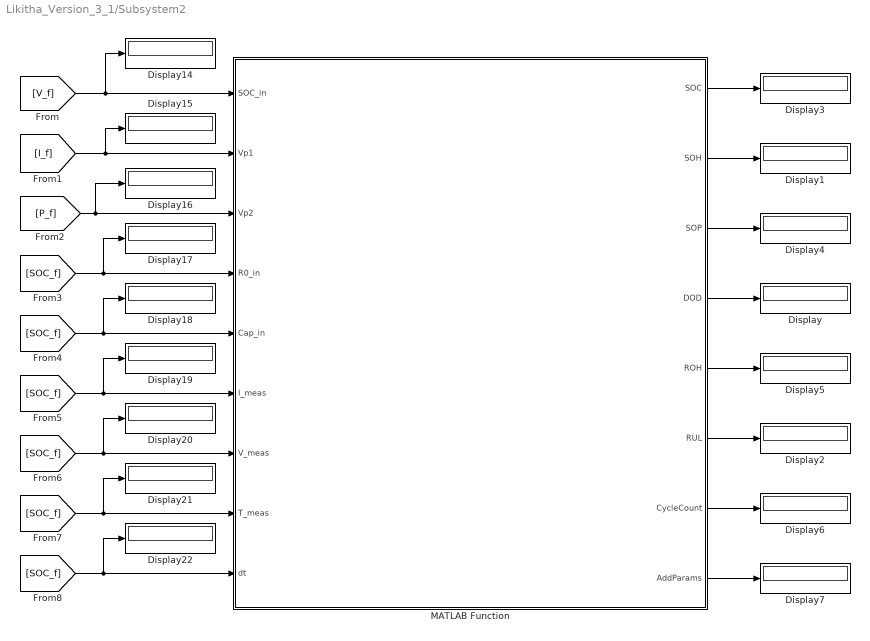
== system Likitha_Version_3_1/Subsystem2 ==
  Display{,1..7,14..22} (17 alike) : Display
  MATLAB Function : MATLAB Function  TreatAsAtomicUnit=on
  wires:
  [V_f] -> MATLAB Function/1(SOC_in), Display14/1
  MATLAB Function/4(DOD) -> Display/1
  MATLAB Function/2(SOH) -> Display1/1
  MATLAB Function/6(RUL) -> Display2/1
  MATLAB Function/1(SOC) -> Display3/1
  MATLAB Function/5(ROH) -> Display5/1
  MATLAB Function/7(CycleCount) -> Display6/1
  MATLAB Function/8(AddParams) -> Display7/1
  MATLAB Function/3(SOP) -> Display4/1
  [I_f] -> MATLAB Function/2(Vp1), Display15/1
  [P_f] -> Display16/1, MATLAB Function/3(Vp2)
  [SOC_f] -> MATLAB Function/4(R0_in), Display17/1
  [SOC_f] -> MATLAB Function/5(Cap_in), Display18/1
  [SOC_f] -> MATLAB Function/6(I_meas), Display19/1
  [SOC_f] -> MATLAB Function/7(V_meas), Display20/1
  [SOC_f] -> MATLAB Function/8(T_meas), Display21/1
  [SOC_f] -> MATLAB Function/9(dt), Display22/1

== system Likitha_Version_3_1/AC to DC/Subsystem1 ==
  Iref : Inport
  Iref* : Inport  Port=2
  Demux : Demux  Outputs=6
  Demux1 : Demux  Outputs=3
  Hysteresis Current Controller (Three-Phase) : eeHysteresisControl/Hysteresis Current Controller (Three-Phase)  h=1  Ts=-1
  Mux : Mux  Inputs=3
  Subsystem : Subsystem
  Terminator{,1..4} (5 alike) : Terminator
  "P14 " : Outport
  P23 : Outport  Port=2
  wires:
  Iref*/1 -> Mux/1
  Subsystem/1(Out1) -> Demux1/1, Hysteresis Current Controller (Three-Phase)/2
  Hysteresis Current Controller (Three-Phase)/1 -> Demux/1
  Demux1/3 -> Mux/3
  Iref/1 -> Subsystem/1(Iref)
  Mux/1 -> Hysteresis Current Controller (Three-Phase)/1
  Demux1/2 -> Mux/2
  Demux/6 -> Terminator4/1
  Demux1/1 -> Terminator/1
  Demux/5 -> Terminator3/1
  Demux/3 -> Terminator1/1
  Demux/4 -> Terminator2/1
  Demux/2 -> P23/1
  Demux/1 -> "P14 "/1

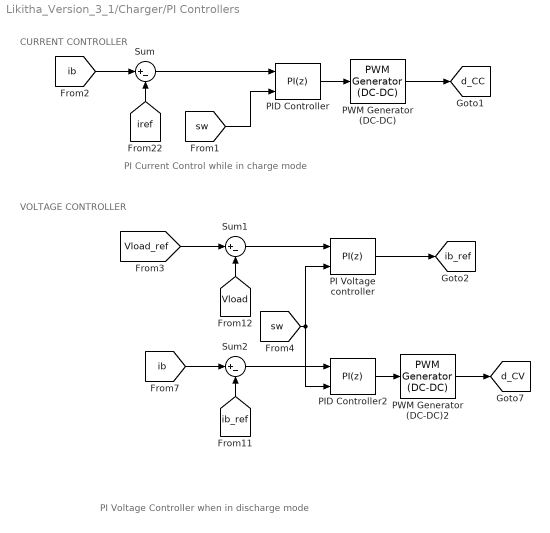
== system Likitha_Version_3_1/Charger/PI Controllers ==
  note: CURRENT CONTROLLER
  note: PI Current Control while in charge mode
  note: VOLTAGE CONTROLLER
  note: PI Voltage Controller when in discharge mode
  PI Voltage controller : slpidlib/PID Controller  Controller=PI  Form=Parallel  TimeDomain=Discrete-time  UseExternalTs=off  SampleTime=500e-6  IntegratorMethod=Forward Euler  FilterMethod=Forward Euler  ControllerParametersSource=internal  P=1  I=10  UseKiTs=off  D=0  UseExternalDerivativeSource=off  N=100  UseFilter=on  TunerSelectOption=Transfer Function Based (PID Tuner App)  InitialConditionSource=internal  InitialConditionForIntegrator=0  InitialConditionForFilter=0  DifferentiatorICPrevScaledInput=0  ExternalReset=falling  TrackingMode=off  Kt=1  LimitOutput=on  SatLimitsSource=internal  UpperSaturationLimit=21.5  LowerSaturationLimit=0  LinearizeAsGain=off  AntiWindupMode=none  Kb=1  LimitIntegrator=off  UpperIntegratorSaturationLimit=inf  LowerIntegratorSaturationLimit=-inf  POutMin=[]  POutMax=[]  IOutMin=[]  IOutMax=[]  DOutMin=[]  DOutMax=[]  NOutMin=[]  NOutMax=[]  SumOutMin=[]  SumOutMax=[]  SaturationOutMin=[]  SaturationOutMax=[]  PParamMin=[]  PParamMax=[]  IParamMin=[]  IParamMax=[]  DParamMin=[]  DParamMax=[]  NParamMin=[]  NParamMax=[]  KbParamMin=[]  KbParamMax=[]  KtParamMin=[]  KtParamMax=[]  KbOutMin=[]  KbOutMax=[]  KtOutMin=[]  KtOutMax=[]  IntegratorOutMin=[]  IntegratorOutMax=[]  FilterOutMin=[]  FilterOutMax=[]  SumI1OutMin=[]  SumI1OutMax=[]  SumI2OutMin=[]  SumI2OutMax=[]  SumI3OutMin=[]  SumI3OutMax=[]  SumI4OutMin=[]  SumI4OutMax=[]  SumDOutMin=[]  SumDOutMax=[]  DifferentiatorOutMin=[]  DifferentiatorOutMax=[]  FilterDiffOutCoefMin=[]  FilterDiffOutCoefMax=[]  ReciprocalOutMin=[]  ReciprocalOutMax=[]  SumDenOutMin=[]  SumDenOutMax=[]  SumNumOutMin=[]  SumNumOutMax=[]  DivideOutMin=[]  DivideOutMax=[]  UdiffTsProdOutMin=[]  UdiffTsProdOutMax=[]  NTsProdOutMin=[]  NTsProdOutMax=[]  UintegralTsProdOutMin=[]  UintegralTsProdOutMax=[]  UngainTsProdOutMin=[]  UngainTsProdOutMax=[]  ClampingZeroOutDataTypeStr=Inherit: Inherit via back propagation  ClampingZeroOutMin=[]  ClampingZeroOutMax=[]  FilterDenConstantOutDataTypeStr=Inherit: Inherit via back propagation  FilterDenConstantOutMin=[]  FilterDenConstantOutMax=[]  PCopyOutDataTypeStr=Inherit: Inherit via back propagation  PCopyOutMin=[]  PCopyOutMax=[]  NCopyOutDataTypeStr=Inherit: Inherit via back propagation  NCopyOutMin=[]  NCopyOutMax=[]  IntegratorContinuousStateAttributes=''  IntegratorStateMustResolveToSignalObject=off  IntegratorRTWStateStorageClass=Auto  FilterContinuousStateAttributes=''  FilterStateMustResolveToSignalObject=off  FilterRTWStateStorageClass=Auto  ParallelPVariant=InternalParameters  IdealPVariant=Disabled  IVariant=InternalParameters  DVariant=Disabled  IntegratorVariant=Discrete  SatVariant=Enabled  AWVariant=Passthrough  PCopyVariant=Disabled  TRVariant=Disabled  FdbkBlocksVariant=Forward  IdealPFdbkVariant=Disabled  SatFdbkVariant=Disabled  DerivativeFilterVariant=Disabled  NVariant=Disabled  NCopyVariant=Disabled_SignalSpec  FilterICVariant=Disabled  IntegratorICVariant=InternalICs  ExternalResetVariant=ExternalReset  TRSumVariant=Passthrough  SumFdbkVariant=Disabled  SumVariant=Sum_PI  TsampFilterVariant=InternalTs  TsampNgainVariant=Passthrough  TsampIntegralVariant=Disabled_SignalSpec  ExternalSaturationOutDataTypeStr=Inherit: Same as second input  DerivativeSourceVariant=Disabled  PreIntVariant=InternalPreInt
  PID Controller : slpidlib/PID Controller  Controller=PI  Form=Parallel  TimeDomain=Discrete-time  UseExternalTs=off  SampleTime=50e-6  IntegratorMethod=Forward Euler  FilterMethod=Forward Euler  ControllerParametersSource=internal  P=0.05  I=10  UseKiTs=off  D=0  UseExternalDerivativeSource=off  N=100  UseFilter=on  TunerSelectOption=Transfer Function Based (PID Tuner App)  InitialConditionSource=internal  InitialConditionForIntegrator=0.54  InitialConditionForFilter=0  DifferentiatorICPrevScaledInput=0  ExternalReset=rising  TrackingMode=off  Kt=1  LimitOutput=on  SatLimitsSource=internal  UpperSaturationLimit=0.95  LowerSaturationLimit=0  LinearizeAsGain=off  AntiWindupMode=none  Kb=1  LimitIntegrator=off  UpperIntegratorSaturationLimit=inf  LowerIntegratorSaturationLimit=-inf  POutMin=[]  POutMax=[]  IOutMin=[]  IOutMax=[]  DOutMin=[]  DOutMax=[]  NOutMin=[]  NOutMax=[]  SumOutMin=[]  SumOutMax=[]  SaturationOutMin=[]  SaturationOutMax=[]  PParamMin=[]  PParamMax=[]  IParamMin=[]  IParamMax=[]  DParamMin=[]  DParamMax=[]  NParamMin=[]  NParamMax=[]  KbParamMin=[]  KbParamMax=[]  KtParamMin=[]  KtParamMax=[]  KbOutMin=[]  KbOutMax=[]  KtOutMin=[]  KtOutMax=[]  IntegratorOutMin=[]  IntegratorOutMax=[]  FilterOutMin=[]  FilterOutMax=[]  SumI1OutMin=[]  SumI1OutMax=[]  SumI2OutMin=[]  SumI2OutMax=[]  SumI3OutMin=[]  SumI3OutMax=[]  SumI4OutMin=[]  SumI4OutMax=[]  SumDOutMin=[]  SumDOutMax=[]  DifferentiatorOutMin=[]  DifferentiatorOutMax=[]  FilterDiffOutCoefMin=[]  FilterDiffOutCoefMax=[]  ReciprocalOutMin=[]  ReciprocalOutMax=[]  SumDenOutMin=[]  SumDenOutMax=[]  SumNumOutMin=[]  SumNumOutMax=[]  DivideOutMin=[]  DivideOutMax=[]  UdiffTsProdOutMin=[]  UdiffTsProdOutMax=[]  NTsProdOutMin=[]  NTsProdOutMax=[]  UintegralTsProdOutMin=[]  UintegralTsProdOutMax=[]  UngainTsProdOutMin=[]  UngainTsProdOutMax=[]  ClampingZeroOutDataTypeStr=Inherit: Inherit via back propagation  ClampingZeroOutMin=[]  ClampingZeroOutMax=[]  FilterDenConstantOutDataTypeStr=Inherit: Inherit via back propagation  FilterDenConstantOutMin=[]  FilterDenConstantOutMax=[]  PCopyOutDataTypeStr=Inherit: Inherit via back propagation  PCopyOutMin=[]  PCopyOutMax=[]  NCopyOutDataTypeStr=Inherit: Inherit via back propagation  NCopyOutMin=[]  NCopyOutMax=[]  IntegratorContinuousStateAttributes=''  IntegratorStateMustResolveToSignalObject=off  IntegratorRTWStateStorageClass=Auto  FilterContinuousStateAttributes=''  FilterStateMustResolveToSignalObject=off  FilterRTWStateStorageClass=Auto  ParallelPVariant=InternalParameters  IdealPVariant=Disabled  IVariant=InternalParameters  DVariant=Disabled  IntegratorVariant=Discrete  SatVariant=Enabled  AWVariant=Passthrough  PCopyVariant=Disabled  TRVariant=Disabled  FdbkBlocksVariant=Forward  IdealPFdbkVariant=Disabled  SatFdbkVariant=Disabled  DerivativeFilterVariant=Disabled  NVariant=Disabled  NCopyVariant=Disabled_SignalSpec  FilterICVariant=Disabled  IntegratorICVariant=InternalICs  ExternalResetVariant=ExternalReset  TRSumVariant=Passthrough  SumFdbkVariant=Disabled  SumVariant=Sum_PI  TsampFilterVariant=InternalTs  TsampNgainVariant=Passthrough  TsampIntegralVariant=Disabled_SignalSpec  ExternalSaturationOutDataTypeStr=Inherit: Same as second input  DerivativeSourceVariant=Disabled  PreIntVariant=InternalPreInt
  PID Controller2 : slpidlib/PID Controller  Controller=PI  Form=Parallel  TimeDomain=Discrete-time  UseExternalTs=off  SampleTime=50e-6  IntegratorMethod=Forward Euler  FilterMethod=Forward Euler  ControllerParametersSource=internal  P=0.05  I=10  UseKiTs=off  D=0  UseExternalDerivativeSource=off  N=100  UseFilter=on  TunerSelectOption=Transfer Function Based (PID Tuner App)  InitialConditionSource=internal  InitialConditionForIntegrator=0.54  InitialConditionForFilter=0  DifferentiatorICPrevScaledInput=0  ExternalReset=falling  TrackingMode=off  Kt=1  LimitOutput=on  SatLimitsSource=internal  UpperSaturationLimit=0.95  LowerSaturationLimit=0  LinearizeAsGain=off  AntiWindupMode=none  Kb=1  LimitIntegrator=off  UpperIntegratorSaturationLimit=inf  LowerIntegratorSaturationLimit=-inf  POutMin=[]  POutMax=[]  IOutMin=[]  IOutMax=[]  DOutMin=[]  DOutMax=[]  NOutMin=[]  NOutMax=[]  SumOutMin=[]  SumOutMax=[]  SaturationOutMin=[]  SaturationOutMax=[]  PParamMin=[]  PParamMax=[]  IParamMin=[]  IParamMax=[]  DParamMin=[]  DParamMax=[]  NParamMin=[]  NParamMax=[]  KbParamMin=[]  KbParamMax=[]  KtParamMin=[]  KtParamMax=[]  KbOutMin=[]  KbOutMax=[]  KtOutMin=[]  KtOutMax=[]  IntegratorOutMin=[]  IntegratorOutMax=[]  FilterOutMin=[]  FilterOutMax=[]  SumI1OutMin=[]  SumI1OutMax=[]  SumI2OutMin=[]  SumI2OutMax=[]  SumI3OutMin=[]  SumI3OutMax=[]  SumI4OutMin=[]  SumI4OutMax=[]  SumDOutMin=[]  SumDOutMax=[]  DifferentiatorOutMin=[]  DifferentiatorOutMax=[]  FilterDiffOutCoefMin=[]  FilterDiffOutCoefMax=[]  ReciprocalOutMin=[]  ReciprocalOutMax=[]  SumDenOutMin=[]  SumDenOutMax=[]  SumNumOutMin=[]  SumNumOutMax=[]  DivideOutMin=[]  DivideOutMax=[]  UdiffTsProdOutMin=[]  UdiffTsProdOutMax=[]  NTsProdOutMin=[]  NTsProdOutMax=[]  UintegralTsProdOutMin=[]  UintegralTsProdOutMax=[]  UngainTsProdOutMin=[]  UngainTsProdOutMax=[]  ClampingZeroOutDataTypeStr=Inherit: Inherit via back propagation  ClampingZeroOutMin=[]  ClampingZeroOutMax=[]  FilterDenConstantOutDataTypeStr=Inherit: Inherit via back propagation  FilterDenConstantOutMin=[]  FilterDenConstantOutMax=[]  PCopyOutDataTypeStr=Inherit: Inherit via back propagation  PCopyOutMin=[]  PCopyOutMax=[]  NCopyOutDataTypeStr=Inherit: Inherit via back propagation  NCopyOutMin=[]  NCopyOutMax=[]  IntegratorContinuousStateAttributes=''  IntegratorStateMustResolveToSignalObject=off  IntegratorRTWStateStorageClass=Auto  FilterContinuousStateAttributes=''  FilterStateMustResolveToSignalObject=off  FilterRTWStateStorageClass=Auto  ParallelPVariant=InternalParameters  IdealPVariant=Disabled  IVariant=InternalParameters  DVariant=Disabled  IntegratorVariant=Discrete  SatVariant=Enabled  AWVariant=Passthrough  PCopyVariant=Disabled  TRVariant=Disabled  FdbkBlocksVariant=Forward  IdealPFdbkVariant=Disabled  SatFdbkVariant=Disabled  DerivativeFilterVariant=Disabled  NVariant=Disabled  NCopyVariant=Disabled_SignalSpec  FilterICVariant=Disabled  IntegratorICVariant=InternalICs  ExternalResetVariant=ExternalReset  TRSumVariant=Passthrough  SumFdbkVariant=Disabled  SumVariant=Sum_PI  TsampFilterVariant=InternalTs  TsampNgainVariant=Passthrough  TsampIntegralVariant=Disabled_SignalSpec  ExternalSaturationOutDataTypeStr=Inherit: Same as second input  DerivativeSourceVariant=Disabled  PreIntVariant=InternalPreInt
  PWM Generator (DC-DC) : spsPWMGeneratorDCDCLib/PWM Generator (DC-DC)  Fsw=10e3  Ts=5e-6
  PWM Generator (DC-DC)2 : spsPWMGeneratorDCDCLib/PWM Generator (DC-DC)  Fsw=10e3  Ts=5e-6
  Sum : Sum  Inputs=|+-
  Sum1 : Sum  Inputs=|+-
  Sum2 : Sum  Inputs=|+-
  tag scope: d_CC=global, d_CV=global, ib_ref=global
  wires:
  [ib] -> Sum/1
  Sum1/1 -> PI Voltage controller/1
  PI Voltage controller/1 -> [ib_ref]
  [ib] -> Sum2/1
  Sum/1 -> PID Controller/1
  PID Controller/1 -> PWM Generator (DC-DC)/1
  [Vload_ref] -> Sum1/1
  [iref] -> Sum/2
  PWM Generator (DC-DC)/1 -> [d_CC]
  PID Controller2/1 -> PWM Generator (DC-DC)2/1
  [Vload] -> Sum1/2
  Sum2/1 -> PID Controller2/1
  [ib_ref] -> Sum2/2
  PWM Generator (DC-DC)2/1 -> [d_CV]
  [sw] -> PID Controller/2
  [sw] -> PI Voltage controller/2, PID Controller2/2

== system Likitha_Version_3_1/Charger/Subsystem ==
  0 current : Constant  Value=0
  Constant : Constant  Value=0
  Multiport Switch : MultiPortSwitch  SaturateOnIntegerOverflow=off  InputSameDT=off
  Multiport Switch1 : MultiPortSwitch  SaturateOnIntegerOverflow=off  InputSameDT=off
  NOT3 : Logic  Operator=NOT  IconShape=distinctive  AllPortsSameDT=off  OutDataTypeStr=boolean
  tag scope: Ref_I=global, s_n=global, s_p=global
  wires:
  Constant/1 -> Multiport Switch/4
  Multiport Switch/1 -> NOT3/1, [s_p]
  NOT3/1 -> [s_n]
  [d_CV] -> Multiport Switch/3
  [d_CC] -> Multiport Switch/2
  [control_cmd] -> Multiport Switch/1
  [iref] -> Multiport Switch1/2
  [ib_ref] -> Multiport Switch1/3
  [control_cmd] -> Multiport Switch1/1
  Multiport Switch1/1 -> [Ref_I]

== system Likitha_Version_3_1/Subsystem/Nref ==
  Add : Sum  Inputs=+++++++
  Step : Step  Time=10  Before=800  After=500  SampleTime=0
  Step1 : Step  Time=20  After=100  SampleTime=0
  Step2 : Step  Time=30  After=100  SampleTime=0
  Step3 : Step  Time=40  After=100  SampleTime=0
  Step4 : Step  Time=50  After=-350  SampleTime=0
  Step5 : Step  Time=60  After=450  SampleTime=0
  Step6 : Step  Time=70  After=100  SampleTime=0
  Out1 : Outport
  wires:
  Step/1 -> Add/1
  Step1/1 -> Add/2
  Step2/1 -> Add/3
  Step3/1 -> Add/4
  Step4/1 -> Add/5
  Step5/1 -> Add/6
  Step6/1 -> Add/7
  Add/1 -> Out1/1
